simulink model "proiect_ep_simulink__version2"  (R2022b)
settings: Solver=FixedStepAuto  StartTime=0.0  StopTime=0.004  FixedStep=1e-5  RelTol=1e-3
values from neighbouring files (symbols this model uses):
  A = 8    [ML.m]
  C = 0.00000519    (= 5.19e-06)    [ML.m]
  Kr = 0.5    [ML.m]
  Ku = 0.48    [ML.m]
  L = 0.01279    [ML.m]
  Rs = 40    [ML.m]
  Rs_20 = 48    [ML.m]
  U21 = 100    [ML.m]
  U21_10 = 110    [ML.m]
libraries: slpidlib x8
settings Model: Creator=nibir  LastModifiedBy=lta

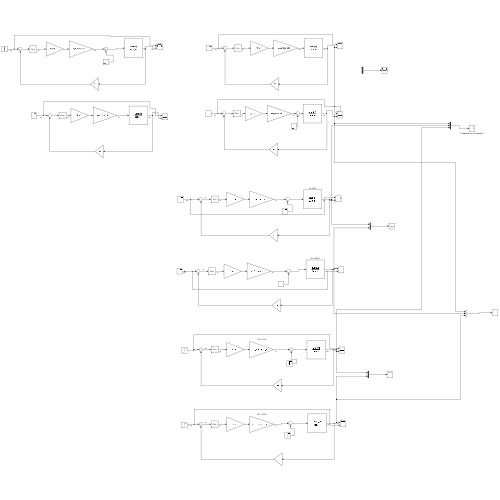
[thumbnail: Simulink's stored preview of the top-level diagram]
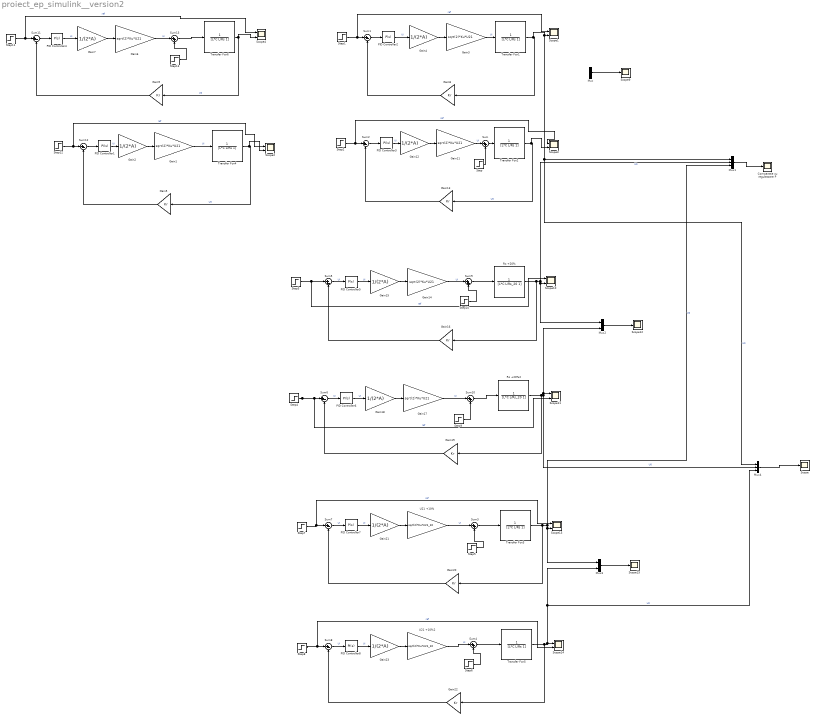
== system proiect_ep_simulink__version2 ==
  Comparatie cu regulatoare P : Scope
  Gain{1,3,6,11,14,17} (6 alike) : Gain  Gain=sqrt(2)*Ku*U21
  Gain{2,4,7,12,15,18,21,23} (8 alike) : Gain  Gain=1/(2*A)
  Gain{5,8..9,13,16,19..20,22} (8 alike) : Gain  Gain=Kr
  Mux : Mux  Inputs=2
  Mux1 : Mux  Inputs=3
  Mux2 : Mux  Inputs=2
  Mux3 : Mux  Inputs=2
  Mux4 : Mux  Inputs=3
  PID Controller{1,3,6,8} (4 alike) : slpidlib/PID Controller  Controller=PI  Form=Parallel  TimeDomain=Continuous-time  UseExternalTs=off  SampleTime=-1  IntegratorMethod=Forward Euler  FilterMethod=Forward Euler  ControllerParametersSource=internal  P=35  I=20  UseKiTs=off  D=0  N=100  UseFilter=on  TunerSelectOption=Transfer Function Based (PID Tuner App)  InitialConditionSource=internal  InitialConditionForIntegrator=0  InitialConditionForFilter=0  DifferentiatorICPrevScaledInput=0  ExternalReset=none  TrackingMode=off  Kt=1  LimitOutput=off  SatLimitsSource=internal  UpperSaturationLimit=inf  LowerSaturationLimit=-inf  LinearizeAsGain=on  AntiWindupMode=none  Kb=1  LimitIntegrator=off  UpperIntegratorSaturationLimit=inf  LowerIntegratorSaturationLimit=-inf  POutMin=[]  POutMax=[]  IOutMin=[]  IOutMax=[]  DOutMin=[]  DOutMax=[]  NOutMin=[]  NOutMax=[]  SumOutMin=[]  SumOutMax=[]  SaturationOutMin=[]  SaturationOutMax=[]  PParamMin=[]  PParamMax=[]  IParamMin=[]  IParamMax=[]  DParamMin=[]  DParamMax=[]  NParamMin=[]  NParamMax=[]  KbParamMin=[]  KbParamMax=[]  KtParamMin=[]  KtParamMax=[]  KbOutMin=[]  KbOutMax=[]  KtOutMin=[]  KtOutMax=[]  IntegratorOutMin=[]  IntegratorOutMax=[]  FilterOutMin=[]  FilterOutMax=[]  SumI1OutMin=[]  SumI1OutMax=[]  SumI2OutMin=[]  SumI2OutMax=[]  SumI3OutMin=[]  SumI3OutMax=[]  SumI4OutMin=[]  SumI4OutMax=[]  SumDOutMin=[]  SumDOutMax=[]  DifferentiatorOutMin=[]  DifferentiatorOutMax=[]  FilterDiffOutCoefMin=[]  FilterDiffOutCoefMax=[]  ReciprocalOutMin=[]  ReciprocalOutMax=[]  SumDenOutMin=[]  SumDenOutMax=[]  SumNumOutMin=[]  SumNumOutMax=[]  DivideOutMin=[]  DivideOutMax=[]  UdiffTsProdOutMin=[]  UdiffTsProdOutMax=[]  NTsProdOutMin=[]  NTsProdOutMax=[]  UintegralTsProdOutMin=[]  UintegralTsProdOutMax=[]  UngainTsProdOutMin=[]  UngainTsProdOutMax=[]  ClampingZeroOutDataTypeStr=Inherit: Inherit via back propagation  ClampingZeroOutMin=[]  ClampingZeroOutMax=[]  FilterDenConstantOutDataTypeStr=Inherit: Inherit via back propagation  FilterDenConstantOutMin=[]  FilterDenConstantOutMax=[]  PCopyOutDataTypeStr=Inherit: Inherit via back propagation  PCopyOutMin=[]  PCopyOutMax=[]  NCopyOutDataTypeStr=Inherit: Inherit via back propagation  NCopyOutMin=[]  NCopyOutMax=[]  IntegratorContinuousStateAttributes=''  IntegratorStateMustResolveToSignalObject=off  IntegratorRTWStateStorageClass=Auto  FilterContinuousStateAttributes=''  FilterStateMustResolveToSignalObject=off  FilterRTWStateStorageClass=Auto  ParallelPVariant=InternalParameters  IdealPVariant=Disabled  IVariant=InternalParameters  DVariant=Disabled  IntegratorVariant=Continuous  SatVariant=Disabled  AWVariant=Passthrough  PCopyVariant=Disabled  TRVariant=Disabled  FdbkBlocksVariant=Forward  IdealPFdbkVariant=Disabled  SatFdbkVariant=Disabled  DerivativeFilterVariant=Disabled  NVariant=Disabled  NCopyVariant=Disabled_SignalSpec  FilterICVariant=Disabled  IntegratorICVariant=InternalICs  ExternalResetVariant=Disabled  TRSumVariant=Passthrough  SumFdbkVariant=Disabled  SumVariant=Sum_PI  TsampFilterVariant=InternalTs  TsampNgainVariant=Passthrough  TsampIntegralVariant=Passthrough  ExternalSaturationOutDataTypeStr=Inherit: Same as second input
  PID Controller{2,4..5,7} (4 alike) : slpidlib/PID Controller  Controller=P  Form=Parallel  TimeDomain=Continuous-time  UseExternalTs=off  SampleTime=-1  IntegratorMethod=Forward Euler  FilterMethod=Forward Euler  ControllerParametersSource=internal  P=35  I=1  UseKiTs=off  D=0  N=100  UseFilter=on  TunerSelectOption=Transfer Function Based (PID Tuner App)  InitialConditionSource=internal  InitialConditionForIntegrator=0  InitialConditionForFilter=0  DifferentiatorICPrevScaledInput=0  ExternalReset=none  TrackingMode=off  Kt=1  LimitOutput=off  SatLimitsSource=internal  UpperSaturationLimit=inf  LowerSaturationLimit=-inf  LinearizeAsGain=on  AntiWindupMode=none  Kb=1  LimitIntegrator=off  UpperIntegratorSaturationLimit=inf  LowerIntegratorSaturationLimit=-inf  POutMin=[]  POutMax=[]  IOutMin=[]  IOutMax=[]  DOutMin=[]  DOutMax=[]  NOutMin=[]  NOutMax=[]  SumOutMin=[]  SumOutMax=[]  SaturationOutMin=[]  SaturationOutMax=[]  PParamMin=[]  PParamMax=[]  IParamMin=[]  IParamMax=[]  DParamMin=[]  DParamMax=[]  NParamMin=[]  NParamMax=[]  KbParamMin=[]  KbParamMax=[]  KtParamMin=[]  KtParamMax=[]  KbOutMin=[]  KbOutMax=[]  KtOutMin=[]  KtOutMax=[]  IntegratorOutMin=[]  IntegratorOutMax=[]  FilterOutMin=[]  FilterOutMax=[]  SumI1OutMin=[]  SumI1OutMax=[]  SumI2OutMin=[]  SumI2OutMax=[]  SumI3OutMin=[]  SumI3OutMax=[]  SumI4OutMin=[]  SumI4OutMax=[]  SumDOutMin=[]  SumDOutMax=[]  DifferentiatorOutMin=[]  DifferentiatorOutMax=[]  FilterDiffOutCoefMin=[]  FilterDiffOutCoefMax=[]  ReciprocalOutMin=[]  ReciprocalOutMax=[]  SumDenOutMin=[]  SumDenOutMax=[]  SumNumOutMin=[]  SumNumOutMax=[]  DivideOutMin=[]  DivideOutMax=[]  UdiffTsProdOutMin=[]  UdiffTsProdOutMax=[]  NTsProdOutMin=[]  NTsProdOutMax=[]  UintegralTsProdOutMin=[]  UintegralTsProdOutMax=[]  UngainTsProdOutMin=[]  UngainTsProdOutMax=[]  ClampingZeroOutDataTypeStr=Inherit: Inherit via back propagation  ClampingZeroOutMin=[]  ClampingZeroOutMax=[]  FilterDenConstantOutDataTypeStr=Inherit: Inherit via back propagation  FilterDenConstantOutMin=[]  FilterDenConstantOutMax=[]  PCopyOutDataTypeStr=Inherit: Inherit via back propagation  PCopyOutMin=[]  PCopyOutMax=[]  NCopyOutDataTypeStr=Inherit: Inherit via back propagation  NCopyOutMin=[]  NCopyOutMax=[]  IntegratorContinuousStateAttributes=''  IntegratorStateMustResolveToSignalObject=off  IntegratorRTWStateStorageClass=Auto  FilterContinuousStateAttributes=''  FilterStateMustResolveToSignalObject=off  FilterRTWStateStorageClass=Auto  ParallelPVariant=InternalParameters  IdealPVariant=Disabled  IVariant=Disabled  DVariant=Disabled  IntegratorVariant=Disabled  SatVariant=Disabled  AWVariant=Disabled  PCopyVariant=Disabled  TRVariant=Disabled  FdbkBlocksVariant=Forward  IdealPFdbkVariant=Disabled  SatFdbkVariant=Disabled  DerivativeFilterVariant=Disabled  NVariant=Disabled  NCopyVariant=Disabled_SignalSpec  FilterICVariant=Disabled  IntegratorICVariant=Disabled  ExternalResetVariant=Disabled  TRSumVariant=Passthrough  SumFdbkVariant=Disabled  SumVariant=Passthrough_P  TsampFilterVariant=InternalTs  TsampNgainVariant=Passthrough  TsampIntegralVariant=Disabled_SignalSpec  ExternalSaturationOutDataTypeStr=Inherit: Same as second input
  Rs +20% : TransferFcn  Denominator=[L*C L/Rs_20 1]
  Rs +20%2 : TransferFcn  Denominator=[L*C L/Rs_20 1]
  Scope{,9,12,15} (4 alike) : Scope
  Scope{1..4,10..11,13..14} (8 alike) : Scope  NumInputPorts=2
  Step{,5..6,9..10,13} (6 alike) : Step  Time=0.0025  After=10  SampleTime=0
  Step{1..4,11..12} (6 alike) : Step  Time=0  Before=1  After=17  SampleTime=1
  Step7 : Step  Time=0  After=17  SampleTime=0
  Step8 : Step  Time=0  After=17  SampleTime=0
  Sum{,3..4,9..10,13} (6 alike) : Sum  Inputs=|++
  Sum{1..2,5..8,11..12} (8 alike) : Sum  Inputs=|+-
  Transfer Fcn{1..6} (6 alike) : TransferFcn  Denominator=[L*C L/Rs 1]
  U21 +10% : Gain  Gain=sqrt(2)*Ku*U21_10
  U21 +10%2 : Gain  Gain=sqrt(2)*Ku*U21_10
  wires:
  Sum1/1 -> PID Controller2/1
  Gain8/1 -> Sum1/2
  Transfer Fcn1/1 -> Mux4/1, Mux1/1, Scope1/2, Gain8/1  "U0"
  Step1/1 -> Scope1/1, Sum1/1  "ref"
  PID Controller2/1 -> Gain4/1  "Ui"
  Gain3/1 -> Transfer Fcn1/1  "Ui"
  Gain4/1 -> Gain3/1
  Gain12/1 -> Gain11/1
  PID Controller3/1 -> Gain12/1  "Ui"
  Transfer Fcn2/1 -> Scope3/2, Gain13/1  "U0"
  Gain13/1 -> Sum2/2
  Step2/1 -> Scope3/1, Sum2/1  "ref"
  Sum2/1 -> PID Controller3/1
  Mux/1 -> Scope9/1
  Gain15/1 -> Gain14/1
  Sum5/1 -> PID Controller5/1  "Ui"
  Gain16/1 -> Sum5/2
  PID Controller5/1 -> Gain15/1  "Ui"
  Step3/1 -> Scope10/1, Sum5/1  "ref"
  PID Controller6/1 -> Gain18/1  "Ui"
  Gain19/1 -> Sum6/2
  Sum6/1 -> PID Controller6/1  "Ui"
  Gain18/1 -> Gain17/1
  Rs +20%2/1 -> Gain19/1, Mux2/2, Scope11/1, Mux4/2  "U0"
  Rs +20%/1 -> Gain16/1, Mux2/1, Scope10/2, Mux1/2  "U0"
  Mux2/1 -> Scope12/1
  Gain21/1 -> U21 +10%/1
  Gain20/1 -> Sum7/2
  PID Controller7/1 -> Gain21/1  "Ui"
  Step7/1 -> Scope13/1, Sum7/1  "ref"
  Sum7/1 -> PID Controller7/1  "Ui"
  Gain22/1 -> Sum8/2
  Gain23/1 -> U21 +10%2/1
  Sum8/1 -> PID Controller8/1  "Ui"
  Step8/1 -> Scope14/2, Sum8/1  "ref"
  PID Controller8/1 -> Gain23/1  "Ui"
  Transfer Fcn5/1 -> Gain22/1, Mux4/3, Mux3/2, Scope14/1  "U0"
  Transfer Fcn3/1 -> Gain20/1, Mux3/1, Scope13/2, Mux1/3  "U0"
  Mux3/1 -> Scope15/1
  Mux1/1 -> Comparatie cu regulatoare P/1
  Mux4/1 -> Scope/1
  Gain11/1 -> Sum/1  "Ui"
  Sum/1 -> Transfer Fcn2/1
  Step/1 -> Sum/2
  Step4/1 -> Scope11/2, Sum6/1  "ref"
  U21 +10%/1 -> Sum3/1  "Ui"
  Sum3/1 -> Transfer Fcn3/1
  Step5/1 -> Sum3/2
  U21 +10%2/1 -> Sum4/1  "Ui"
  Sum4/1 -> Transfer Fcn5/1
  Step6/1 -> Sum4/2
  Gain17/1 -> Sum10/1  "Ui"
  Sum10/1 -> Rs +20%2/1
  Gain14/1 -> Sum9/1  "Ui"
  Sum9/1 -> Rs +20%/1
  Step9/1 -> Sum10/2
  Step10/1 -> Sum9/2
  Sum12/1 -> PID Controller1/1
  Step12/1 -> Scope2/1, Sum12/1  "ref"
  Gain2/1 -> Gain1/1
  Transfer Fcn4/1 -> Scope2/2, Gain5/1  "U0"
  Gain5/1 -> Sum12/2
  PID Controller1/1 -> Gain2/1  "Ui"
  Gain1/1 -> Transfer Fcn4/1  "Ui"
  Gain7/1 -> Gain6/1
  Gain9/1 -> Sum11/2
  PID Controller4/1 -> Gain7/1  "Ui"
  Step11/1 -> Scope4/1, Sum11/1  "ref"
  Transfer Fcn6/1 -> Scope4/2, Gain9/1  "U0"
  Sum11/1 -> PID Controller4/1
  Gain6/1 -> Sum13/1  "Ui"
  Sum13/1 -> Transfer Fcn6/1
  Step13/1 -> Sum13/2
